simulink model "PID_Motor_Controller"  (R2020a)
settings: Solver=VariableStepAuto  StartTime=0.0  StopTime=15  RelTol=1e-3
settings Model: Creator=Rizve Chowdhury  LastModifiedBy=Rizve Chowdhury
settings SolverCC: ZeroCrossAlgorithm=Adaptive  AlgebraicLoopSolver=LineSearch
settings DebuggingCC: IgnoredZcDiagnostic=none

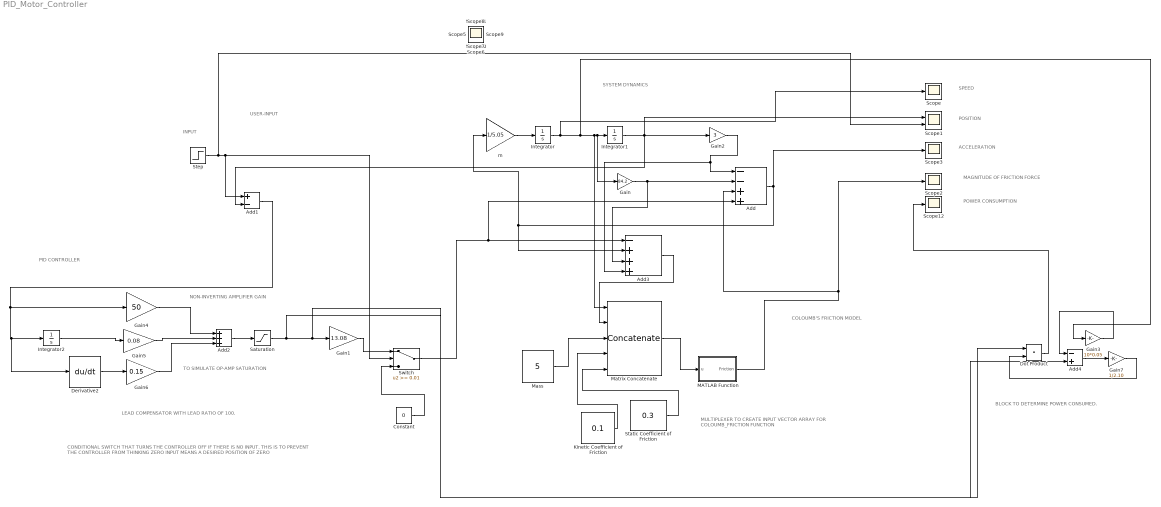
== system PID_Motor_Controller ==
  note: POWER CONSUMPTION
  note: BLOCK TO DETERMINE
      | POWER CONSUMED.
  note: CONDITIONAL SWITCH THAT TURNS THE CONTROLLER OFF
      | IF THERE IS NO INPUT. THIS IS TO PREVENT THE CONTROLLER
      | FROM THINKING ZERO INPUT MEANS A DESIRED POSITION OF ZERO
  note: SYSTEM DYNAMICS
  note: USER-INPUT
  note: ACCELERATION
  note: POSITION
  note: SPEED
  note: MULTIPLEXER TO CREATE
      | INPUT VECTOR ARRAY FOR
      | COLOUMB_FRICTION FUNCTION
  note: COLOUMB'S FRICTION MODEL
  note: MAGNITUDE OF FRICTION FORCE
  note: LEAD COMPENSATOR WITH
      | LEAD RATIO OF 100.
  note: PID CONTROLLER
  note: TO SIMULATE OP-AMP SATURATION
  note: INPUT
  note: NON-INVERTING AMPLIFIER GAIN
  Add : Sum  Inputs=--++
  Add1 : Sum  Inputs=+-
  Add2 : Sum  Inputs=3
  Add3 : Sum  Inputs=-+++
  Add4 : Sum  Inputs=-+
  Constant : Constant  Value=0
  Derivative2 : Derivative  CoefficientInTFapproximation=0.01
  Dot Product : DotProduct  InputSameDT=on  OutDataTypeStr=Inherit: Inherit via internal rule
  Gain : Gain  Gain=84.2
  Gain1 : Gain  Gain=13.08
  Gain2 : Gain  Gain=3
  Gain3 : Gain  Gain=10*0.05
  Gain4 : Gain  Gain=50
  Gain5 : Gain  Gain=0.08
  Gain6 : Gain  Gain=0.15
  Gain7 : Gain  Gain=1/2.10
  Integrator : Integrator
  Integrator1 : Integrator  InitialCondition=0.5
  Integrator2 : Integrator
  Kinetic Coefficient of Friction : Constant  Value=0.1
  MATLAB Function : MATLAB Function  TreatAsAtomicUnit=on
  Mass : Constant  Value=5
  Matrix Concatenate : Concatenate  NumInputs=5  ConcatenateDimension=2
  Saturation : Saturate  UpperLimit=5  LowerLimit=-5
  Scope{,2..12} (12 alike) : Scope
  Scope1 : Scope  NumInputPorts=2
  Static Coefficient of Friction : Constant  Value=0.3
  Step : Step  After=0.3  SampleTime=0
  Switch : Switch  Threshold=0.01
  m : Gain  Gain=1/5.05
  wires:
  Gain/1 -> Add3/3, Add/2
  Gain2/1 -> Add3/4, Add/1
  Static Coefficient of Friction/1 -> Matrix Concatenate/5
  Matrix Concatenate/1 -> MATLAB Function/1(u)
  Mass/1 -> Matrix Concatenate/3
  Kinetic Coefficient of Friction/1 -> Matrix Concatenate/4
  MATLAB Function/1(Friction) -> Add/3, Scope2/1
  m/1 -> Integrator/1
  Gain6/1 -> Add2/3
  Integrator2/1 -> Gain5/1
  Gain5/1 -> Add2/2
  Derivative2/1 -> Gain6/1
  Integrator/1 -> Scope/1, Gain3/1, Matrix Concatenate/1, Gain/1, Integrator1/1
  Gain4/1 -> Add2/1
  Integrator1/1 -> Add1/2, Scope1/1, Gain2/1
  Step/1 -> Switch/2, Add1/1, Scope1/2
  Add1/1 -> Gain4/1, Derivative2/1, Integrator2/1
  Add/1 -> m/1, Add3/2, Scope3/1
  Add2/1 -> Saturation/1
  Add3/1 -> Matrix Concatenate/2
  Constant/1 -> Switch/3
  Gain1/1 -> Switch/1
  Switch/1 -> Add/4, Add3/1
  Dot Product/1 -> Scope12/1
  Gain3/1 -> Add4/1
  Saturation/1 -> Add4/2, Dot Product/1, Gain1/1
  Add4/1 -> Gain7/1
  Gain7/1 -> Dot Product/2

== matlab function PID_Motor_Controller/MATLAB Function ==
  data: u input; Friction output
function Friction = Colomb_Friction(u)
%The input u is a 6-tuple
%u(1) is the velocity
%u(2) is the net force
%u(3) is the mass
%u(4) is the kinetic coefficient of friction
%u(5) is the static coefficient of friction
speed = u(1);
TOL = 1E-3;
if (length(u) > 1)
    Static_Friction = u(5)*u(3)*9.8;
    Kinetic_Friction = u(4)*u(3)*9.8;
    Net_Force = u(2);
    if (abs(speed) < TOL)
        if (abs(Net_Force) < Static_Friction)
        Friction = -Net_Force; 
        else
        Friction = -Kinetic_Friction*sign(u(1));  
        end
    else
        Friction = -Kinetic_Friction*sign(u(1));
    end
else
    Friction = 0;
end
